simulink model "ADEL"  (R2024a)
settings: Solver=ode45  StartTime=0.0  StopTime=7  MaxStep=1e-5  RelTol=1e-3  EnableMultiTasking=on
values from neighbouring files (symbols this model uses):
  G = zpk([-10], [0 -2], [5])    [tp2.m]
  Ts = .09    (= 0.09)    [tp2.m]
undefined symbols (not defined in the file or in its folder): ADEL
settings Model: Creator=Usuario  LastModifiedBy=Clifferto
settings SolverCC: AlgebraicLoopSolver=TrustRegion
settings DataIOCC: SaveFormat=Array  SignalLoggingSaveFormat=ModelDataLogs  ReturnWorkspaceOutputs=off
settings OptimizationCC: InitFltsAndDblsToZero=on  LifeSpan=inf
settings DebuggingCC: SaveWithParameterizedLinksMsg=none  UnderspecifiedInitializationDetection=Classic  MergeDetectMultiDrivingBlocksExec=none  SignalResolutionControl=TryResolveAllWithWarning  SolverPrmCheckMsg=warning  MultiTaskDSMMsg=warning  MultiTaskCondExecSysMsg=none  FcnCallInpInsideContextMsg=warning  UnconnectedInputMsg=warning  UnconnectedOutputMsg=warning  UnconnectedLineMsg=warning  SFUnexpectedBacktrackingDiag=warning  SFNoUnconditionalDefaultTransitionDiag=warning  SFExecutionAtInitializationDiag=none  ArithmeticOperatorsInVariantConditions=warning
settings HardwareCC: ProdBitPerPointer=32  ProdBitPerSizeT=32  ProdBitPerPtrDiffT=32  ProdLargestAtomicFloat=None  ProdIntDivRoundTo=Undefined  ProdEndianess=Unspecified  ProdWordSize=32  ProdHWDeviceType=32-bit Generic
settings ModelReferenceCC: PropagateSignalLabelsOutOfModel=off
settings SFSimCC: SimUseLocalCustomCode=off  CustomCodeUndefinedFunction=UseInterfaceOnly
settings RTWCC: RTWUseLocalCustomCode=off  GPUComputeCapability=3.5
settings CodeAppCC: StateflowObjectComments=on
settings GRTTargetCC: TargetFcnLib=ansi_tfl_tmw.mat  TargetLangStandard=C89/C90 (ANSI)  CombineOutputUpdateFcns=off  GRTInterface=on
settings ConfigComp: CovMetricSettings=dw  CovSaveCumulativeToWorkspaceVar=on  CovSaveSingleToWorkspaceVar=on  CovExternalEMLEnable=off  CovSFcnEnable=off

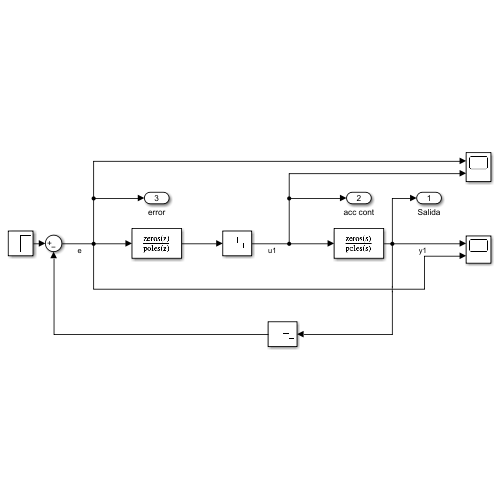
[thumbnail: Simulink's stored preview of the top-level diagram]
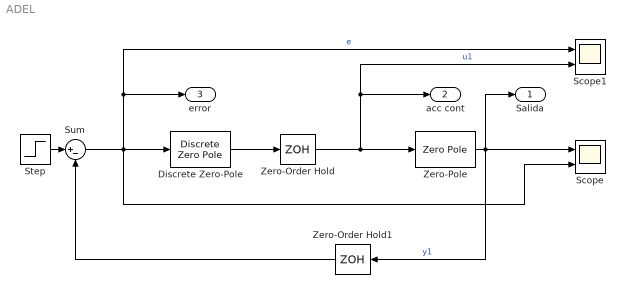
== system ADEL ==
  Discrete Zero-Pole : DiscreteZeroPole  Zeros=ADEL.Z{:}  Poles=ADEL.P{:}  Gain=ADEL.K  SampleTime=-1
  Scope : Scope  NumInputPorts=2
  Scope1 : Scope  NumInputPorts=2
  Step : Step  Time=0  SampleTime=Ts
  Sum : Sum  Inputs=|+-
  Zero-Order Hold : ZeroOrderHold  SampleTime=Ts
  Zero-Order Hold1 : ZeroOrderHold  SampleTime=Ts
  Zero-Pole : ZeroPole  Zeros=G.Z{:}  Poles=G.P{:}  Gain=G.K
  Salida : Outport
  acc cont : Outport  Port=2
  error : Outport  Port=3
  wires:
  Zero-Order Hold/1 -> Zero-Pole/1, acc cont/1, Scope1/2  "u1"
  Step/1 -> Sum/1
  Zero-Pole/1 -> Zero-Order Hold1/1, Scope/1, Salida/1  "y1"
  Zero-Order Hold1/1 -> Sum/2
  Sum/1 -> Scope1/1, error/1, Scope/2, Discrete Zero-Pole/1  "e"
  Discrete Zero-Pole/1 -> Zero-Order Hold/1
